simulink model "integralImage_hdl_2018b"  (R2018b)
settings: Solver=FixedStepDiscrete  StartTime=0.0  StopTime=totalPixels  RelTol=1e-3
InitFcn:
  | frm2pix = visionhdl.FrameToPixels;
  | frm2pix.VideoFormat = '240p';
  | [activePixelsPerLine, activeLines, totalPixels] = getparamfromfrm2pix(frm2pix);
undefined symbols (not defined in the file or in its folder): activePixelsPerLine, totalPixels
libraries: visionhdlio x1, hdlsllib x1, visionsources x1
settings Model: SimulationMode=accelerator  Creator=linbai  LastModifiedBy=linbai
settings DataIOCC: ReturnWorkspaceOutputs=on
settings HardwareCC: ProdBitPerPointer=32  ProdBitPerSizeT=32  ProdBitPerPtrDiffT=32  ProdLargestAtomicFloat=None  ProdIntDivRoundTo=Undefined  ProdEndianess=Unspecified  ProdWordSize=32  ProdHWDeviceType=ASIC/FPGA->ASIC/FPGA  TargetBitPerPointer=64  TargetBitPerSizeT=64  TargetBitPerPtrDiffT=64  TargetLongLongMode=on  TargetIntDivRoundTo=Zero  TargetEndianess=LittleEndian  TargetWordSize=64  TargetHWDeviceType=Custom Processor->MATLAB Host Computer  ProdEqTarget=off

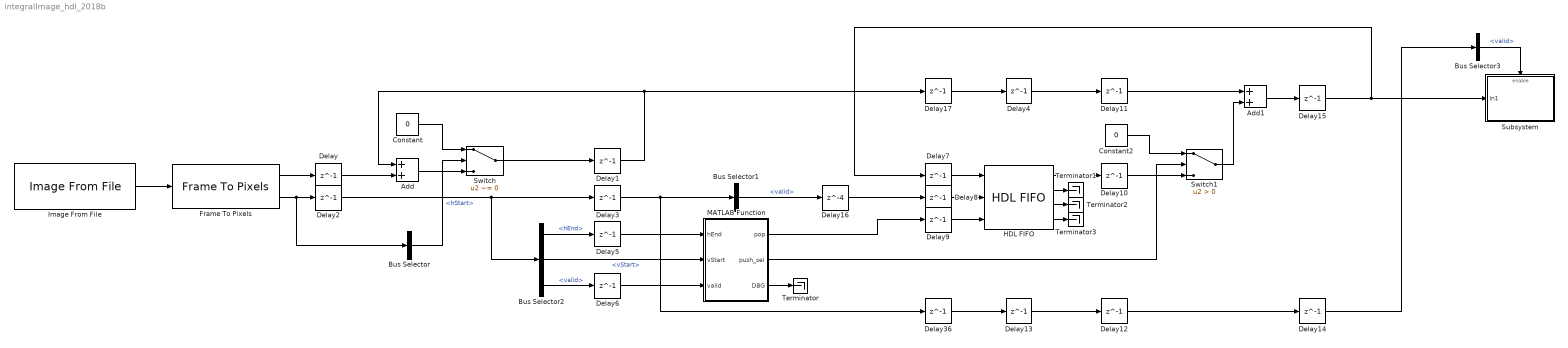
== system integralImage_hdl_2018b ==
  Add : Sum  OutDataTypeStr=fixdt(0,nextpow2(255*activePixelsPerLine*activeLines),0)
  Add1 : Sum  OutDataTypeStr=fixdt(0,nextpow2(255*activePixelsPerLine*activeLines),0)
  Bus Selector : BusSelector  OutputSignals=hStart
  Bus Selector1 : BusSelector  OutputSignals=valid
  Bus Selector2 : BusSelector  OutputSignals=hEnd,vStart,valid
  Bus Selector3 : BusSelector  OutputSignals=valid
  Constant : Constant  Value=0  OutDataTypeStr=uint8  SampleTime=-1
  Constant2 : Constant  Value=0  OutDataTypeStr=uint8  SampleTime=-1
  Delay{,1..15,17,36} (18 alike) : Delay  DelayLength=1
  Delay16 : Delay  DelayLength=4
  Frame To Pixels : visionhdlio/Frame To Pixels  NumComponents=1  NumPixels=1  VideoFormat=240p  ActivePixelsPerLine=160  ActiveVideoLines=160  TotalPixelsPerLine=400  TotalVideoLines=400  StartingActiveLine=6  FrontPorch=120  SampleTime=0
      settings: SourceProductName=Vision HDL Toolbox  SourceProductBaseCode=VT
  HDL FIFO : hdlsllib/HDL RAMs/HDL FIFO  fifo_size=2^(nextpow2(activePixelsPerLine))  mode=Classic  ratio=1  push_msg=Warning  pop_msg=Warning  show_empty=on  show_full=on  show_num=on  LabelModeActiveChoice_Mode=Classic
      settings: SourceProductName=Simulink  SourceProductBaseCode=SL
  Image From File : visionsources/Image From File  Tag=vipblks_nd  FileName=.\img_test.png  Ts=totalPixels  imagePorts=One multidimensional signal  OutPortLabels=R|G|B  ImageDataType=Inherit from input image  sdImageDataType=uint(8)  Signed=on  WordLength=16  FractionLengthMode=User-defined  FractionLength=15
      settings: SourceProductName=Computer Vision Toolbox
  MATLAB Function : MATLAB Function  TreatAsAtomicUnit=on
  Subsystem : Subsystem
  Switch : Switch  Criteria=u2 ~= 0
  Switch1 : Switch  Criteria=u2 > Threshold
  Terminator{,1..3} (4 alike) : Terminator
  wires:
  Image From File/1 -> Frame To Pixels/1
  Delay/1 -> Add/2
  Frame To Pixels/1 -> Delay/1
  Add/1 -> Switch/3
  Constant/1 -> Switch/1
  Delay2/1 -> Bus Selector2/1, Delay3/1
  Frame To Pixels/2 -> Bus Selector/1, Delay2/1
  Bus Selector/1 -> Switch/2  "<hStart>"
  HDL FIFO/1 -> Delay10/1
  MATLAB Function/3(DBG) -> Terminator/1
  Bus Selector2/1 -> Delay5/1  "<hEnd>"
  Bus Selector2/2 -> MATLAB Function/2(vStart)  "<vStart>"
  Bus Selector2/3 -> Delay6/1  "<valid>"
  Delay6/1 -> MATLAB Function/3(valid)
  Delay5/1 -> MATLAB Function/1(hEnd)
  Delay7/1 -> HDL FIFO/1
  Delay8/1 -> HDL FIFO/2
  Delay9/1 -> HDL FIFO/3
  Delay4/1 -> Delay11/1
  Delay11/1 -> Add1/1
  Add1/1 -> Delay15/1
  Delay13/1 -> Delay12/1
  Delay12/1 -> Delay14/1
  Delay14/1 -> Bus Selector3/1
  Bus Selector3/1 -> Subsystem/Enable  "<valid>"
  Switch/1 -> Delay1/1
  HDL FIFO/2 -> Terminator1/1
  HDL FIFO/3 -> Terminator2/1
  HDL FIFO/4 -> Terminator3/1
  MATLAB Function/1(pop) -> Delay9/1
  Switch1/1 -> Add1/2
  Delay10/1 -> Switch1/3
  Constant2/1 -> Switch1/1
  MATLAB Function/2(push_sel) -> Switch1/2
  Delay16/1 -> Delay8/1
  Delay15/1 -> Subsystem/1(In1), Delay7/1
  Bus Selector1/1 -> Delay16/1  "<valid>"
  Delay3/1 -> Bus Selector1/1, Delay36/1
  Delay1/1 -> Add/1, Delay17/1
  Delay17/1 -> Delay4/1
  Delay36/1 -> Delay13/1

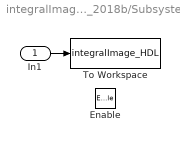
== system integralImage_hdl_2018b/Subsystem ==
  In1 : Inport
  Enable : EnablePort
  To Workspace : ToWorkspace  VariableName=integralImage_HDL  SaveFormat=Timeseries  SampleTime=-1
  wires:
  In1/1 -> To Workspace/1

== matlab function integralImage_hdl_2018b/MATLAB Function ==
  data: pop output; push_sel output; hEnd input; vStart input; valid input; DBG output
function [pop, push_sel, DBG] = fcn(hEnd, vStart, valid)

S0_NORMAL  = ufi(0,2,0);
S1_NON_POP = ufi(1,2,0);

% using persistent keyword to model state registers in hardware
persistent curr_state;
if isempty(curr_state)
    curr_state = S0_NORMAL;   
end

switch curr_state
    case S0_NORMAL
        pop = valid;
        push_sel = false;
        curr_state = S0_NORMAL;
        
        if vStart
            curr_state = S1_NON_POP;
        else
            
        end
        
    case S1_NON_POP
        pop = false;
        push_sel = true;
        curr_state = S1_NON_POP;
        
        if hEnd
            curr_state = S0_NORMAL;
        end
        
    otherwise
        pop = false;
        push_sel = false;
        curr_state = S0_NORMAL;
end

DBG = curr_state;
